simulink model "test_flocking_algorithm"  (R2025b)
settings: Solver=ode4  StartTime=0.0  StopTime=200  FixedStep=0.1  RelTol=1e-3
InitFcn:
  | % initialization_2d
values from neighbouring files (symbols this model uses):
  d2r = 0.0174532925199    [DDPG_HybridFlocking_agents8-4-1.mat]    (also in flocking_learning.m; initialization_2d.m)
  g = spec(2)    [ActualOutput.m]    (also in DDPG_HybridFlocking_agents8-4-1.mat = 9.806; ModelSwarm.m; initialization.m = 9.806; initialization_2d.m = 9.806)
  m = spec(1)    [ActualOutput.m]    (also in DDPG_HybridFlocking_agents8-4-1.mat = 5; ModelSwarm.m; initialization.m = 15; initialization_2d.m = 5)
  state0 = [435.012620465 721.15936685 20 2.59881408791 0 187.945467124 786.05177403 20 2.90689824266 0 842.493878094 376.880931214 ... (25 elements, 5x5)]    [DDPG_HybridFlocking_agents8-4-1.mat]    (also in flocking_learning.m = zeros(5, N); initialization.m = [x0; y0; z0; V0; gam0; psi0]; initialization_2d.m = [x0; y0; V0; psi0; bank0])
undefined symbols (not defined in the file or in its folder): init_state
libraries: simulink_extras x10, rllib x6
(part 1 of 2)
settings Model: Creator=chang  LastModifiedBy=laaa

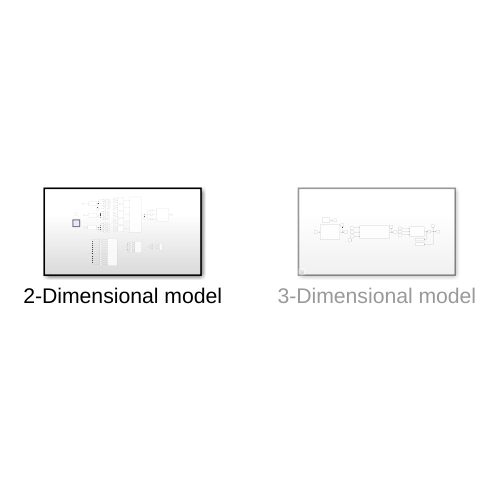
[thumbnail: Simulink's stored preview of the top-level diagram]
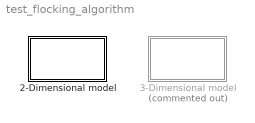
== system test_flocking_algorithm ==
  2-Dimensional model : Subsystem
  3-Dimensional model : Subsystem  Commented=on

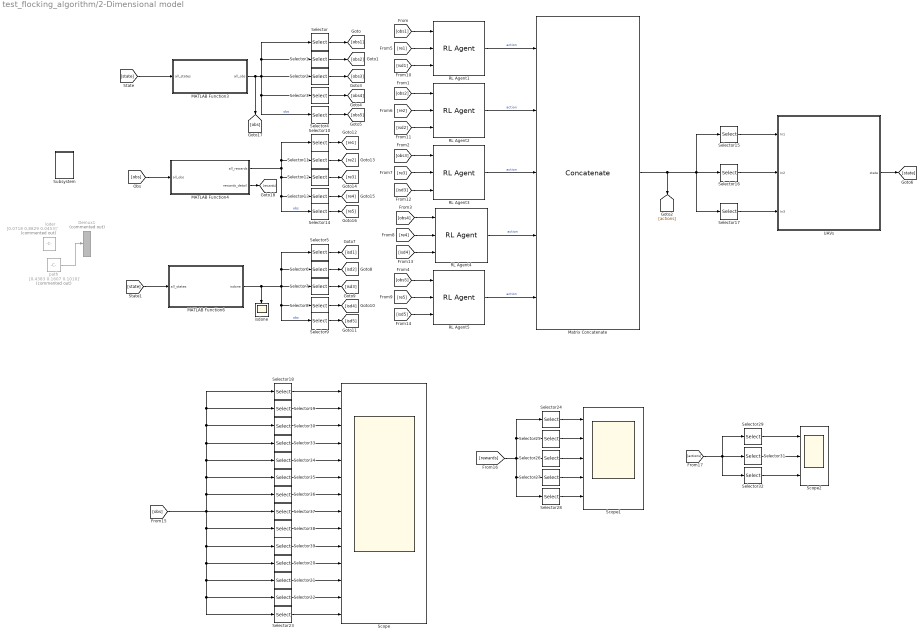
== system test_flocking_algorithm/2-Dimensional model ==
  Demux1 : Demux  Commented=on  Outputs=3
  MATLAB Function3 : MATLAB Function  TreatAsAtomicUnit=on
  MATLAB Function4 : MATLAB Function  TreatAsAtomicUnit=on
  MATLAB Function6 : MATLAB Function  TreatAsAtomicUnit=on
  Matrix Concatenate : Concatenate  NumInputs=5  Mode=Multidimensional array  ConcatenateDimension=2
  RL Agent1 : rllib/RL Agent  Agent=agentObj1  ExternalActionAsInput=off  ProvideLastAction=off  ProvideCumRwd=off  TreatAsDirectFeedthrough=on  UseStrictObservationDataTypes=off
  RL Agent2 : rllib/RL Agent  Agent=agentObj2  ExternalActionAsInput=off  ProvideLastAction=off  ProvideCumRwd=off  TreatAsDirectFeedthrough=on  UseStrictObservationDataTypes=off
  RL Agent3 : rllib/RL Agent  Agent=agentObj3  ExternalActionAsInput=off  ProvideLastAction=off  ProvideCumRwd=off  TreatAsDirectFeedthrough=on  UseStrictObservationDataTypes=off
  RL Agent4 : rllib/RL Agent  Agent=agentObj4  ExternalActionAsInput=off  ProvideLastAction=off  ProvideCumRwd=off  TreatAsDirectFeedthrough=on  UseStrictObservationDataTypes=off
  RL Agent5 : rllib/RL Agent  Agent=agentObj5  ExternalActionAsInput=off  ProvideLastAction=off  ProvideCumRwd=off  TreatAsDirectFeedthrough=on  UseStrictObservationDataTypes=off
  Scope : Scope  NumInputPorts=14
      settings: TimeSpan=200  ActiveDisplayString=12  ShowGrid=off  ActiveDisplayYMinimum=-1.9279504121774151  ActiveDisplayYMaximum=1.9179370597420149  DataLoggingVariableName=ScopeData11
  Scope1 : Scope  NumInputPorts=5
      settings: TimeSpan=200  ActiveDisplayString=5  ShowGrid=off  ActiveDisplayYMinimum=0.0009  ActiveDisplayYMaximum=0.0011  DataLoggingVariableName=ScopeData25
  Scope2 : Scope  NumInputPorts=3
      settings: TimeSpan=200  ActiveDisplayString=3  ShowGrid=off  ActiveDisplayYMinimum=-1  ActiveDisplayYMaximum=1  DataLoggingVariableName=ScopeData26
  Selector : Selector  NumberOfDimensions=2  InputPortWidth=3  IndexOptions=Index vector (dialog),Index vector (dialog)  Indices=1:14,1  OutputSizes=1,1
  Selector1 : Selector  NumberOfDimensions=2  InputPortWidth=3  IndexOptions=Index vector (dialog),Index vector (dialog)  Indices=1:14,2  OutputSizes=1,1
  Selector10 : Selector  NumberOfDimensions=2  InputPortWidth=3  IndexOptions=Index vector (dialog),Index vector (dialog)  Indices=1,1  OutputSizes=1,1
  Selector11 : Selector  NumberOfDimensions=2  InputPortWidth=3  IndexOptions=Index vector (dialog),Index vector (dialog)  Indices=1,2  OutputSizes=1,1
  Selector12 : Selector  NumberOfDimensions=2  InputPortWidth=3  IndexOptions=Index vector (dialog),Index vector (dialog)  Indices=1,3  OutputSizes=1,1
  Selector13 : Selector  NumberOfDimensions=2  InputPortWidth=3  IndexOptions=Index vector (dialog),Index vector (dialog)  Indices=1,4  OutputSizes=1,1
  Selector14 : Selector  NumberOfDimensions=2  InputPortWidth=3  IndexOptions=Index vector (dialog),Index vector (dialog)  Indices=1,5  OutputSizes=1,1
  Selector{15,18,24,29} (4 alike) : Selector  NumberOfDimensions=2  InputPortWidth=3  IndexOptions=Index vector (dialog),Index vector (dialog)  Indices=1,1:5  OutputSizes=1,1
  Selector{16,19,25,31} (4 alike) : Selector  NumberOfDimensions=2  InputPortWidth=3  IndexOptions=Index vector (dialog),Index vector (dialog)  Indices=2,1:5  OutputSizes=1,1
  Selector{17,26,30,32} (4 alike) : Selector  NumberOfDimensions=2  InputPortWidth=3  IndexOptions=Index vector (dialog),Index vector (dialog)  Indices=3,1:5  OutputSizes=1,1
  Selector2 : Selector  NumberOfDimensions=2  InputPortWidth=3  IndexOptions=Index vector (dialog),Index vector (dialog)  Indices=1:14,3  OutputSizes=1,1
  Selector20 : Selector  NumberOfDimensions=2  InputPortWidth=3  IndexOptions=Index vector (dialog),Index vector (dialog)  Indices=11,1:5  OutputSizes=1,1
  Selector21 : Selector  NumberOfDimensions=2  InputPortWidth=3  IndexOptions=Index vector (dialog),Index vector (dialog)  Indices=12,1:5  OutputSizes=1,1
  Selector22 : Selector  NumberOfDimensions=2  InputPortWidth=3  IndexOptions=Index vector (dialog),Index vector (dialog)  Indices=13,1:5  OutputSizes=1,1
  Selector23 : Selector  NumberOfDimensions=2  InputPortWidth=3  IndexOptions=Index vector (dialog),Index vector (dialog)  Indices=14,1:5  OutputSizes=1,1
  Selector27 : Selector  NumberOfDimensions=2  InputPortWidth=3  IndexOptions=Index vector (dialog),Index vector (dialog)  Indices=4,1:5  OutputSizes=1,1
  Selector28 : Selector  NumberOfDimensions=2  InputPortWidth=3  IndexOptions=Index vector (dialog),Index vector (dialog)  Indices=5,1:5  OutputSizes=1,1
  Selector3 : Selector  NumberOfDimensions=2  InputPortWidth=3  IndexOptions=Index vector (dialog),Index vector (dialog)  Indices=1:14,4  OutputSizes=1,1
  Selector33 : Selector  NumberOfDimensions=2  InputPortWidth=3  IndexOptions=Index vector (dialog),Index vector (dialog)  Indices=4,1:5  OutputSizes=1,1
  Selector34 : Selector  NumberOfDimensions=2  InputPortWidth=3  IndexOptions=Index vector (dialog),Index vector (dialog)  Indices=5,1:5  OutputSizes=1,1
  Selector35 : Selector  NumberOfDimensions=2  InputPortWidth=3  IndexOptions=Index vector (dialog),Index vector (dialog)  Indices=6,1:5  OutputSizes=1,1
  Selector36 : Selector  NumberOfDimensions=2  InputPortWidth=3  IndexOptions=Index vector (dialog),Index vector (dialog)  Indices=7,1:5  OutputSizes=1,1
  Selector37 : Selector  NumberOfDimensions=2  InputPortWidth=3  IndexOptions=Index vector (dialog),Index vector (dialog)  Indices=8,1:5  OutputSizes=1,1
  Selector38 : Selector  NumberOfDimensions=2  InputPortWidth=3  IndexOptions=Index vector (dialog),Index vector (dialog)  Indices=9,1:5  OutputSizes=1,1
  Selector39 : Selector  NumberOfDimensions=2  InputPortWidth=3  IndexOptions=Index vector (dialog),Index vector (dialog)  Indices=10,1:5  OutputSizes=1,1
  Selector4 : Selector  NumberOfDimensions=2  InputPortWidth=3  IndexOptions=Index vector (dialog),Index vector (dialog)  Indices=1:14,5  OutputSizes=1,1
  Selector5 : Selector  NumberOfDimensions=2  InputPortWidth=3  IndexOptions=Index vector (dialog),Index vector (dialog)  Indices=1,1  OutputSizes=1,1
  Selector6 : Selector  NumberOfDimensions=2  InputPortWidth=3  IndexOptions=Index vector (dialog),Index vector (dialog)  Indices=1,2  OutputSizes=1,1
  Selector7 : Selector  NumberOfDimensions=2  InputPortWidth=3  IndexOptions=Index vector (dialog),Index vector (dialog)  Indices=1,3  OutputSizes=1,1
  Selector8 : Selector  NumberOfDimensions=2  InputPortWidth=3  IndexOptions=Index vector (dialog),Index vector (dialog)  Indices=1,4  OutputSizes=1,1
  Selector9 : Selector  NumberOfDimensions=2  InputPortWidth=3  IndexOptions=Index vector (dialog),Index vector (dialog)  Indices=1,5  OutputSizes=1,1
  Subsystem : Subsystem
  UAVs : Subsystem
  isdone : Scope
      settings: TimeSpan=300  ActiveDisplayYMinimum=-1  ActiveDisplayYMaximum=1  DataLoggingVariableName=ScopeData23
  loiter : Constant  Commented=on  Value=[0.0718 0.8829 0.0453]'
  path : Constant  Commented=on  Value=[0.4383 0.1607 0.1010]'
  wires:
  Selector4/1 -> [obs5]
  Selector7/1 -> [isd3]
  [re1] -> RL Agent1/2
  [re4] -> RL Agent4/2
  RL Agent1/1 -> Matrix Concatenate/1  "action"
  [isd3] -> RL Agent3/3
  [isd5] -> RL Agent5/3
  RL Agent2/1 -> Matrix Concatenate/2  "action"
  path/1 -> Demux1/1
  [isd2] -> RL Agent2/3
  Selector10/1 -> [re1]
  RL Agent4/1 -> Matrix Concatenate/4  "action"
  Selector17/1 -> UAVs/3(In3)
  Selector8/1 -> [isd4]
  Selector5/1 -> [isd1]
  MATLAB Function6/1(isdone) -> Selector5/1, Selector6/1, Selector7/1, Selector8/1, Selector9/1, isdone/1  "obs"
  [state] -> MATLAB Function6/1(all_states)
  Selector16/1 -> UAVs/2(In2)
  Selector9/1 -> [isd5]
  Selector13/1 -> [re4]
  [obs2] -> RL Agent2/1
  MATLAB Function4/2(rewards_detail) -> [rewards]
  [obs] -> MATLAB Function4/1(all_obs)
  [re3] -> RL Agent3/2
  [obs1] -> RL Agent1/1
  UAVs/1(state) -> [state]
  RL Agent5/1 -> Matrix Concatenate/5  "action"
  Selector3/1 -> [obs4]
  [re2] -> RL Agent2/2
  Selector6/1 -> [isd2]
  [isd1] -> RL Agent1/3
  Selector14/1 -> [re5]
  Selector11/1 -> [re2]
  Selector2/1 -> [obs3]
  MATLAB Function3/1(all_obs) -> Selector2/1, Selector3/1, Selector4/1, Selector/1, Selector1/1, [obs]  "obs"
  Selector1/1 -> [obs2]
  [isd4] -> RL Agent4/3
  Matrix Concatenate/1 -> [actions], Selector16/1, Selector15/1, Selector17/1
  [re5] -> RL Agent5/2
  Selector12/1 -> [re3]
  [obs4] -> RL Agent4/1
  MATLAB Function4/1(all_rewards) -> Selector12/1, Selector13/1, Selector14/1, Selector10/1, Selector11/1  "obs"
  RL Agent3/1 -> Matrix Concatenate/3  "action"
  Selector15/1 -> UAVs/1(In1)
  [obs3] -> RL Agent3/1
  [state] -> MATLAB Function3/1(all_states)
  Selector/1 -> [obs1]
  [obs5] -> RL Agent5/1
  Selector22/1 -> Scope/13
  Selector19/1 -> Scope/2
  Selector36/1 -> Scope/7
  Selector30/1 -> Scope/3
  Selector25/1 -> Scope1/2
  Selector34/1 -> Scope/5
  Selector32/1 -> Scope2/3
  Selector33/1 -> Scope/4
  Selector37/1 -> Scope/8
  Selector26/1 -> Scope1/3
  [actions] -> Selector32/1, Selector29/1, Selector31/1
  Selector38/1 -> Scope/9
  [rewards] -> Selector28/1, Selector27/1, Selector25/1, Selector24/1, Selector26/1
  Selector20/1 -> Scope/11
  Selector24/1 -> Scope1/1
  Selector18/1 -> Scope/1
  [obs] -> Selector39/1, Selector20/1, Selector21/1, Selector23/1, Selector22/1, Selector38/1, Selector33/1, Selector30/1, Selector19/1, Selector18/1, Selector34/1, Selector35/1, Selector36/1, Selector37/1
  Selector23/1 -> Scope/14
  Selector29/1 -> Scope2/1
  Selector27/1 -> Scope1/4
  Selector28/1 -> Scope1/5
  Selector39/1 -> Scope/10
  Selector35/1 -> Scope/6
  Selector31/1 -> Scope2/2
  Selector21/1 -> Scope/12

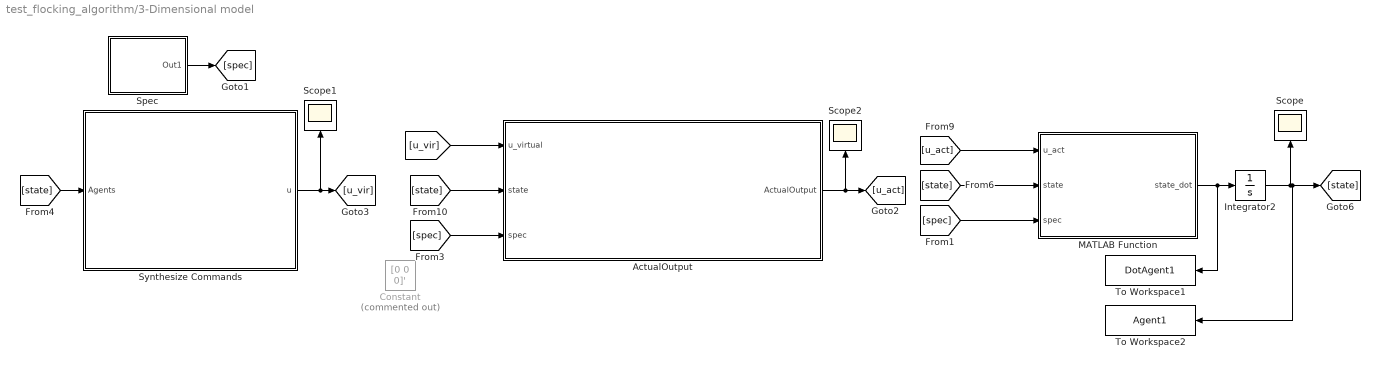
== system test_flocking_algorithm/3-Dimensional model ==
  ActualOutput : Subsystem
  Constant : Constant  Commented=on  Value=[0 0 0]'
  Integrator2 : Integrator  InitialCondition=state0  UpperSaturationLimit=[10^6 ;10^6 ;10^6 ;30 ;15 ;10^6]  LowerSaturationLimit=[-10^6; -10^6 ;-10^6; 0; -15 ;-10^6]'
  MATLAB Function : MATLAB Function  TreatAsAtomicUnit=on
  Scope : Scope
      settings: ActiveDisplayYMinimum=-1796.4442274835574  ActiveDisplayYMaximum=1827.1129411617226
  Scope1 : Scope
      settings: ActiveDisplayYMinimum=-0.625  ActiveDisplayYMaximum=0.625
  Scope2 : Scope
      settings: ActiveDisplayYMinimum=-543.50698903671855  ActiveDisplayYMaximum=2400.6247544411835  DataLoggingVariableName=ScopeData2
  Spec : Subsystem
  Synthesize Commands : Subsystem
  To Workspace1 : ToWorkspace  VariableName=DotAgent1  SaveFormat=Timeseries  SampleTime=-1
  To Workspace2 : ToWorkspace  VariableName=Agent1  SaveFormat=Timeseries  SampleTime=-1
  wires:
  [spec] -> MATLAB Function/3(spec)
  Synthesize Commands/1(u) -> Scope1/1, [u_vir]
  [state] -> ActualOutput/2(state)
  [spec] -> ActualOutput/3(spec)
  [state] -> Synthesize Commands/1(Agents)
  Integrator2/1 -> [state], To Workspace2/1, Scope/1
  [u_vir] -> ActualOutput/1(u_virtual)
  ActualOutput/1(ActualOutput) -> Scope2/1, [u_act]
  MATLAB Function/1(state_dot) -> To Workspace1/1, Integrator2/1
  Spec/1(Out1) -> [spec]
  [state] -> MATLAB Function/2(state)
  [u_act] -> MATLAB Function/1(u_act)

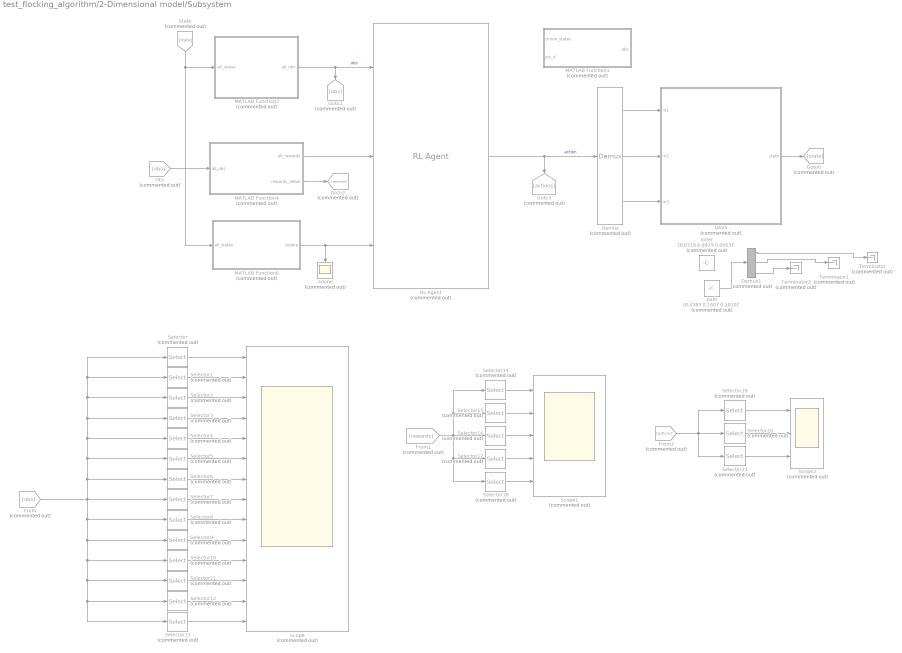
== system test_flocking_algorithm/2-Dimensional model/Subsystem ==
  Demux : Demux  Commented=on  Outputs=3
  Demux1 : Demux  Commented=on  Outputs=3
  From : From  Commented=on  GotoTag=obs
  From1 : From  Commented=on  GotoTag=rewards
  From2 : From  Commented=on  GotoTag=actions
  Goto1 : Goto  Commented=on  GotoTag=obs
  Goto2 : Goto  Commented=on  GotoTag=rewards
  Goto3 : Goto  Commented=on  GotoTag=actions
  Goto6 : Goto  Commented=on  GotoTag=state
  MATLAB Function1 : MATLAB Function  Commented=on  TreatAsAtomicUnit=on
  MATLAB Function3 : MATLAB Function  Commented=on  TreatAsAtomicUnit=on
  MATLAB Function4 : MATLAB Function  Commented=on  TreatAsAtomicUnit=on
  MATLAB Function6 : MATLAB Function  Commented=on  TreatAsAtomicUnit=on
  Obs : From  Commented=on  GotoTag=obs
  RL Agent : rllib/RL Agent  Commented=on  Agent=agent  ExternalActionAsInput=off  ProvideLastAction=off  ProvideCumRwd=off  TreatAsDirectFeedthrough=on  UseStrictObservationDataTypes=off
  Scope : Scope  Commented=on  NumInputPorts=14
      settings: DataLoggingVariableName=ScopeData15
  Scope1 : Scope  Commented=on  NumInputPorts=5
      settings: DataLoggingVariableName=ScopeData17
  Scope2 : Scope  Commented=on  NumInputPorts=3
      settings: DataLoggingVariableName=ScopeData20
  Selector : Selector  Commented=on  NumberOfDimensions=2  InputPortWidth=3  IndexOptions=Index vector (dialog),Index vector (dialog)  Indices=1,1:5  OutputSizes=1,1
  Selector1 : Selector  Commented=on  NumberOfDimensions=2  InputPortWidth=3  IndexOptions=Index vector (dialog),Index vector (dialog)  Indices=2,1:5  OutputSizes=1,1
  Selector10 : Selector  Commented=on  NumberOfDimensions=2  InputPortWidth=3  IndexOptions=Index vector (dialog),Index vector (dialog)  Indices=11,1:5  OutputSizes=1,1
  Selector11 : Selector  Commented=on  NumberOfDimensions=2  InputPortWidth=3  IndexOptions=Index vector (dialog),Index vector (dialog)  Indices=12,1:5  OutputSizes=1,1
  Selector12 : Selector  Commented=on  NumberOfDimensions=2  InputPortWidth=3  IndexOptions=Index vector (dialog),Index vector (dialog)  Indices=13,1:5  OutputSizes=1,1
  Selector13 : Selector  Commented=on  NumberOfDimensions=2  InputPortWidth=3  IndexOptions=Index vector (dialog),Index vector (dialog)  Indices=14,1:5  OutputSizes=1,1
  Selector14 : Selector  Commented=on  NumberOfDimensions=2  InputPortWidth=3  IndexOptions=Index vector (dialog),Index vector (dialog)  Indices=1,1:5  OutputSizes=1,1
  Selector15 : Selector  Commented=on  NumberOfDimensions=2  InputPortWidth=3  IndexOptions=Index vector (dialog),Index vector (dialog)  Indices=2,1:5  OutputSizes=1,1
  Selector16 : Selector  Commented=on  NumberOfDimensions=2  InputPortWidth=3  IndexOptions=Index vector (dialog),Index vector (dialog)  Indices=3,1:5  OutputSizes=1,1
  Selector17 : Selector  Commented=on  NumberOfDimensions=2  InputPortWidth=3  IndexOptions=Index vector (dialog),Index vector (dialog)  Indices=4,1:5  OutputSizes=1,1
  Selector18 : Selector  Commented=on  NumberOfDimensions=2  InputPortWidth=3  IndexOptions=Index vector (dialog),Index vector (dialog)  Indices=5,1:5  OutputSizes=1,1
  Selector19 : Selector  Commented=on  NumberOfDimensions=2  InputPortWidth=3  IndexOptions=Index vector (dialog),Index vector (dialog)  Indices=1,1:5  OutputSizes=1,1
  Selector2 : Selector  Commented=on  NumberOfDimensions=2  InputPortWidth=3  IndexOptions=Index vector (dialog),Index vector (dialog)  Indices=3,1:5  OutputSizes=1,1
  Selector20 : Selector  Commented=on  NumberOfDimensions=2  InputPortWidth=3  IndexOptions=Index vector (dialog),Index vector (dialog)  Indices=2,1:5  OutputSizes=1,1
  Selector21 : Selector  Commented=on  NumberOfDimensions=2  InputPortWidth=3  IndexOptions=Index vector (dialog),Index vector (dialog)  Indices=3,1:5  OutputSizes=1,1
  Selector3 : Selector  Commented=on  NumberOfDimensions=2  InputPortWidth=3  IndexOptions=Index vector (dialog),Index vector (dialog)  Indices=4,1:5  OutputSizes=1,1
  Selector4 : Selector  Commented=on  NumberOfDimensions=2  InputPortWidth=3  IndexOptions=Index vector (dialog),Index vector (dialog)  Indices=5,1:5  OutputSizes=1,1
  Selector5 : Selector  Commented=on  NumberOfDimensions=2  InputPortWidth=3  IndexOptions=Index vector (dialog),Index vector (dialog)  Indices=6,1:5  OutputSizes=1,1
  Selector6 : Selector  Commented=on  NumberOfDimensions=2  InputPortWidth=3  IndexOptions=Index vector (dialog),Index vector (dialog)  Indices=7,1:5  OutputSizes=1,1
  Selector7 : Selector  Commented=on  NumberOfDimensions=2  InputPortWidth=3  IndexOptions=Index vector (dialog),Index vector (dialog)  Indices=8,1:5  OutputSizes=1,1
  Selector8 : Selector  Commented=on  NumberOfDimensions=2  InputPortWidth=3  IndexOptions=Index vector (dialog),Index vector (dialog)  Indices=9,1:5  OutputSizes=1,1
  Selector9 : Selector  Commented=on  NumberOfDimensions=2  InputPortWidth=3  IndexOptions=Index vector (dialog),Index vector (dialog)  Indices=10,1:5  OutputSizes=1,1
  State : From  Commented=on  GotoTag=state
  Terminator : Terminator  Commented=on
  Terminator1 : Terminator  Commented=on
  Terminator2 : Terminator  Commented=on
  UAVs : Subsystem  Commented=on
  isdone : Scope  Commented=on
      settings: TimeSpan=300  ActiveDisplayYMinimum=-1  ActiveDisplayYMaximum=1  DataLoggingVariableName=ScopeData12
  loiter : Constant  Commented=on  Value=[0.0718 0.8829 0.0453]'
  path : Constant  Commented=on  Value=[0.4383 0.1607 0.1010]'
  wires:
  From/1 -> Selector9/1, Selector10/1, Selector11/1, Selector13/1, Selector12/1, Selector8/1, Selector3/1, Selector2/1, Selector1/1, Selector/1, Selector4/1, Selector5/1, Selector6/1, Selector7/1
  Demux/1 -> UAVs/1(In1)
  MATLAB Function3/1(all_obs) -> Goto1/1, RL Agent/1  "obs"
  Selector11/1 -> Scope/12
  Selector10/1 -> Scope/11
  Selector14/1 -> Scope1/1
  Demux/2 -> UAVs/2(In2)
  Obs/1 -> MATLAB Function4/1(all_obs)
  State/1 -> MATLAB Function6/1(all_states), MATLAB Function3/1(all_states)
  From1/1 -> Selector18/1, Selector17/1, Selector15/1, Selector14/1, Selector16/1
  Selector5/1 -> Scope/6
  Selector19/1 -> Scope2/1
  Selector16/1 -> Scope1/3
  Demux1/1 -> Terminator/1
  Selector18/1 -> Scope1/5
  Selector9/1 -> Scope/10
  From2/1 -> Selector21/1, Selector19/1, Selector20/1
  path/1 -> Demux1/1
  RL Agent/1 -> Goto3/1, Demux/1  "action"
  Selector3/1 -> Scope/4
  Selector21/1 -> Scope2/3
  UAVs/1(state) -> Goto6/1
  MATLAB Function6/1(isdone) -> RL Agent/3, isdone/1
  MATLAB Function4/1(all_rewards) -> RL Agent/2
  Selector/1 -> Scope/1
  Demux/3 -> UAVs/3(In3)
  Selector8/1 -> Scope/9
  Selector7/1 -> Scope/8
  Selector6/1 -> Scope/7
  Selector15/1 -> Scope1/2
  Selector2/1 -> Scope/3
  Demux1/3 -> Terminator2/1
  Demux1/2 -> Terminator1/1
  Selector17/1 -> Scope1/4
  Selector20/1 -> Scope2/2
  Selector12/1 -> Scope/13
  Selector13/1 -> Scope/14
  MATLAB Function4/2(rewards_detail) -> Goto2/1
  Selector1/1 -> Scope/2
  Selector4/1 -> Scope/5

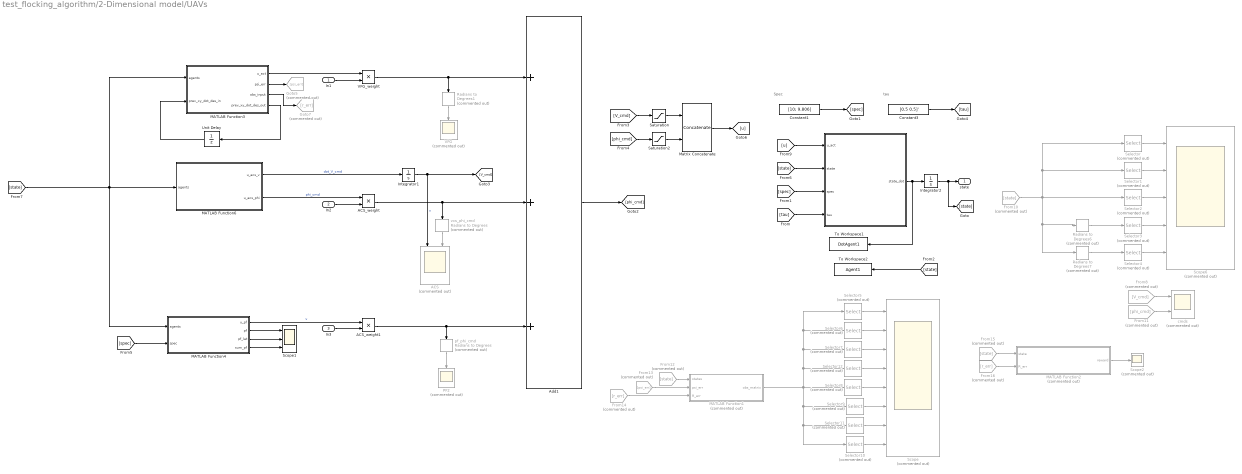
== system test_flocking_algorithm/2-Dimensional model/UAVs ==
  note: Spec
  note: tau
  In1 : Inport
  In2 : Inport  Port=2
  In3 : Inport  Port=3
  " " : MATLAB Function  TreatAsAtomicUnit=on
  ACS : Scope  Commented=on  NumInputPorts=2
      settings: ActiveDisplayYMinimum=-23.869601726691815  ActiveDisplayYMaximum=64.370407175335345  DataLoggingVariableName=ScopeData9
  ACS_weight : Product
  ACS_weight1 : Product
  Add1 : Sum  Inputs=+++
  Constant1 : Constant  Value=[10; 9.806]
  Constant3 : Constant  Value=[0.5 0.5]'
  From10 : From  Commented=on  GotoTag=state
  From11 : From  Commented=on  GotoTag=phi_cmd
  From12 : From  Commented=on  GotoTag=state
  From13 : From  Commented=on  GotoTag=psi_err
  From14 : From  Commented=on  GotoTag=r_err
  From15 : From  Commented=on  GotoTag=state
  From16 : From  Commented=on  GotoTag=r_err
  From8 : From  Commented=on  GotoTag=V_cmd
  Goto5 : Goto  Commented=on  GotoTag=psi_err
  Goto7 : Goto  Commented=on  GotoTag=r_err
  Integrator1 : Integrator  LimitOutput=on  UpperSaturationLimit=35*ones(1,5)  LowerSaturationLimit=15*ones(1,5)
  Integrator2 : Integrator  InitialCondition=init_state  LimitOutput=on  UpperSaturationLimit=[10^6; 10^6; 35; 10^6; 30*d2r ].*ones(1,5)  LowerSaturationLimit=[-10^6; -10^6; 15; -10^6; -30*d2r ].*ones(1,5)
  MATLAB Function1 : MATLAB Function  Commented=on  TreatAsAtomicUnit=on
  MATLAB Function2 : MATLAB Function  Commented=on  TreatAsAtomicUnit=on
  MATLAB Function3 : MATLAB Function  TreatAsAtomicUnit=on
  MATLAB Function4 : MATLAB Function  TreatAsAtomicUnit=on
  MATLAB Function6 : MATLAB Function  TreatAsAtomicUnit=on
  Matrix Concatenate : Concatenate  Mode=Multidimensional array
  PF2 : Scope  Commented=on
      settings: TimeSpan=300  ActiveDisplayYMinimum=-44.741397355611163  ActiveDisplayYMaximum=44.744942341518566  DataLoggingVariableName=ScopeData10
  Radians to Degrees1 : simulink_extras/Transformations/Radians to Degrees  Commented=on
  Radians to Degrees6 : simulink_extras/Transformations/Radians to Degrees  Commented=on
  Radians to Degrees7 : simulink_extras/Transformations/Radians to Degrees  Commented=on
  Saturation : Saturate  UpperLimit=35*ones(1,5)  LowerLimit=15*ones(1,5)
  Saturation2 : Saturate  UpperLimit=30*d2r*ones(1,5)  LowerLimit=-30*d2r*ones(1,5)  LinearizeAsGain=off
  Scope : Scope  Commented=on  NumInputPorts=8
      settings: ActiveDisplayString=4  ActiveDisplayYMinimum=0.29571525373676022  ActiveDisplayYMaximum=1.0782538606959156  DataLoggingVariableName=ScopeData18
  Scope1 : Scope  NumInputPorts=3
      settings: ActiveDisplayYMinimum=-1  ActiveDisplayYMaximum=1  DataLoggingVariableName=ScopeData16
  Scope2 : Scope  Commented=on
      settings: ActiveDisplayYMinimum=-109.38583360755611  ActiveDisplayYMaximum=7.8590338705691378  DataLoggingVariableName=ScopeData19
  Scope6 : Scope  Commented=on  NumInputPorts=5
      settings: TimeSpan=300  ActiveDisplayString=5  ShowGrid=off  ActiveDisplayYMinimum=-37.354494394302066  ActiveDisplayYMaximum=37.435243344907619  YLabel=Bank angle (deg)  DataLoggingVariableName=ScopeData13
  Selector : Selector  Commented=on  NumberOfDimensions=2  InputPortWidth=3  IndexOptions=Index vector (dialog),Index vector (dialog)  Indices=1,1:10  OutputSizes=1,1
  Selector1 : Selector  Commented=on  NumberOfDimensions=2  InputPortWidth=3  IndexOptions=Index vector (dialog),Index vector (dialog)  Indices=2,1:10  OutputSizes=1,1
  Selector10 : Selector  Commented=on  NumberOfDimensions=2  InputPortWidth=3  IndexOptions=Index vector (dialog),Index vector (dialog)  Indices=8,1:5  OutputSizes=1,1
  Selector11 : Selector  Commented=on  NumberOfDimensions=2  InputPortWidth=3  IndexOptions=Index vector (dialog),Index vector (dialog)  Indices=7,1:5  OutputSizes=1,1
  Selector12 : Selector  Commented=on  NumberOfDimensions=2  InputPortWidth=3  IndexOptions=Index vector (dialog),Index vector (dialog)  Indices=4,1:5  OutputSizes=1,1
  Selector2 : Selector  Commented=on  NumberOfDimensions=2  InputPortWidth=3  IndexOptions=Index vector (dialog),Index vector (dialog)  Indices=3,1:10  OutputSizes=1,1
  Selector3 : Selector  Commented=on  NumberOfDimensions=2  InputPortWidth=3  IndexOptions=Index vector (dialog),Index vector (dialog)  Indices=4,1:10  OutputSizes=1,1
  Selector4 : Selector  Commented=on  NumberOfDimensions=2  InputPortWidth=3  IndexOptions=Index vector (dialog),Index vector (dialog)  Indices=5,1:10  OutputSizes=1,1
  Selector5 : Selector  Commented=on  NumberOfDimensions=2  InputPortWidth=3  IndexOptions=Index vector (dialog),Index vector (dialog)  Indices=1,1:5  OutputSizes=1,1
  Selector6 : Selector  Commented=on  NumberOfDimensions=2  InputPortWidth=3  IndexOptions=Index vector (dialog),Index vector (dialog)  Indices=2,1:5  OutputSizes=1,1
  Selector7 : Selector  Commented=on  NumberOfDimensions=2  InputPortWidth=3  IndexOptions=Index vector (dialog),Index vector (dialog)  Indices=3,1:5  OutputSizes=1,1
  Selector8 : Selector  Commented=on  NumberOfDimensions=2  InputPortWidth=3  IndexOptions=Index vector (dialog),Index vector (dialog)  Indices=5,1:5  OutputSizes=1,1
  Selector9 : Selector  Commented=on  NumberOfDimensions=2  InputPortWidth=3  IndexOptions=Index vector (dialog),Index vector (dialog)  Indices=6,1:5  OutputSizes=1,1
  To Workspace1 : ToWorkspace  VariableName=DotAgent1  SaveFormat=Timeseries  SampleTime=-1
  To Workspace2 : ToWorkspace  VariableName=Agent1  SaveFormat=Timeseries  SampleTime=-1
  Unit Delay : UnitDelay  SampleTime=-1  HasFrameUpgradeWarning=on
  VFG : Scope  Commented=on
      settings: ActiveDisplayYMinimum=-2.2311275771009429  ActiveDisplayYMaximum=1.6680942354459041  DataLoggingVariableName=ScopeData8
  VFG_weight : Product
  cmds : Scope  Commented=on  NumInputPorts=2
      settings: ActiveDisplayYMinimum=-0.21104649012249277  ActiveDisplayYMaximum=0.44117626715669322  DataLoggingVariableName=ScopeData14
  pf_phi_cmd : simulink_extras/Transformations/Radians to Degrees  Commented=on
  vcs_phi_cmd : simulink_extras/Transformations/Radians to Degrees  Commented=on
  state : Outport
  wires:
  " "/1(state_dot) -> To Workspace1/1, Integrator2/1
  [state] -> MATLAB Function4/1(agents), MATLAB Function3/1(agents), MATLAB Function6/1(agents)
  [spec] -> MATLAB Function4/2(spec)
  MATLAB Function4/1(u_pf) -> ACS_weight1/1  "v"
  MATLAB Function6/2(u_acs_phi) -> ACS_weight/1  "phi_cmd"
  MATLAB Function3/1(u_act) -> VFG_weight/1
  In1/1 -> VFG_weight/2
  VFG_weight/1 -> Radians to Degrees1/1, Add1/1
  Radians to Degrees1/1 -> VFG/1
  MATLAB Function6/1(u_acs_v) -> Integrator1/1  "dot_V_cmd"
  Integrator1/1 -> ACS/1, [V_cmd]  "v"
  ACS_weight/1 -> Add1/2, vcs_phi_cmd/1
  In2/1 -> ACS_weight/2
  vcs_phi_cmd/1 -> ACS/2
  MATLAB Function4/4(sum_pf) -> Scope1/3
  MATLAB Function4/3(pf_lat) -> Scope1/2
  MATLAB Function4/2(pf) -> Scope1/1
  In3/1 -> ACS_weight1/2
  ACS_weight1/1 -> pf_phi_cmd/1, Add1/3
  pf_phi_cmd/1 -> PF2/1
  Add1/1 -> [phi_cmd]
  [V_cmd] -> Saturation/1
  [phi_cmd] -> Saturation2/1
  Saturation/1 -> Matrix Concatenate/1
  Saturation2/1 -> Matrix Concatenate/2
  Matrix Concatenate/1 -> [u]
  [u] -> " "/1(u_act)
  [state] -> " "/2(state)
  [spec] -> " "/3(spec)
  [tau] -> " "/4(tau)
  Constant1/1 -> [spec]
  Constant3/1 -> [tau]
  Integrator2/1 -> [state], state/1
  [state] -> To Workspace2/1
  Selector/1 -> Scope6/1
  Selector1/1 -> Scope6/2
  Selector2/1 -> Scope6/3
  Selector3/1 -> Scope6/4
  Selector4/1 -> Scope6/5
  From10/1 -> Selector2/1, Selector/1, Selector1/1, Radians to Degrees6/1, Radians to Degrees7/1
  Radians to Degrees6/1 -> Selector3/1
  Radians to Degrees7/1 -> Selector4/1
  From8/1 -> cmds/1
  From11/1 -> cmds/2
  MATLAB Function3/2(psi_err) -> Goto5/1
  MATLAB Function3/3(obs_input) -> Goto7/1
  From12/1 -> MATLAB Function1/1(states)
  From13/1 -> MATLAB Function1/2(psi_err)
  From14/1 -> MATLAB Function1/3(R_err)
  MATLAB Function1/1(obs_matrix) -> Selector6/1, Selector5/1, Selector7/1, Selector12/1, Selector8/1, Selector9/1, Selector10/1, Selector11/1
  Selector9/1 -> Scope/6
  Selector11/1 -> Scope/7
  Selector10/1 -> Scope/8
  Selector5/1 -> Scope/1
  Selector6/1 -> Scope/2
  Selector7/1 -> Scope/3
  Selector12/1 -> Scope/4
  Selector8/1 -> Scope/5
  From15/1 -> MATLAB Function2/1(state)
  From16/1 -> MATLAB Function2/2(R_err)
  MATLAB Function2/1(reward) -> Scope2/1
  MATLAB Function3/4(prev_xy_dot_des_out) -> Unit Delay/1
  Unit Delay/1 -> MATLAB Function3/2(prev_xy_dot_des_in)

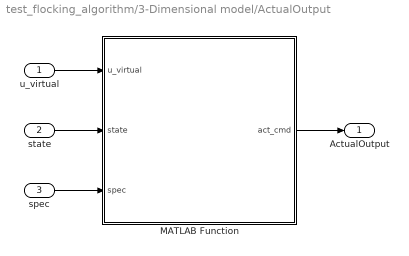
== system test_flocking_algorithm/3-Dimensional model/ActualOutput ==
  u_virtual : Inport
  state : Inport  Port=2
  spec : Inport  Port=3
  MATLAB Function : MATLAB Function  TreatAsAtomicUnit=on
  ActualOutput : Outport
  wires:
  u_virtual/1 -> MATLAB Function/1(u_virtual)
  state/1 -> MATLAB Function/2(state)
  spec/1 -> MATLAB Function/3(spec)
  MATLAB Function/1(act_cmd) -> ActualOutput/1

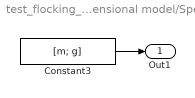
== system test_flocking_algorithm/3-Dimensional model/Spec ==
  Constant3 : Constant  Value=[m; g]
  Out1 : Outport
  wires:
  Constant3/1 -> Out1/1

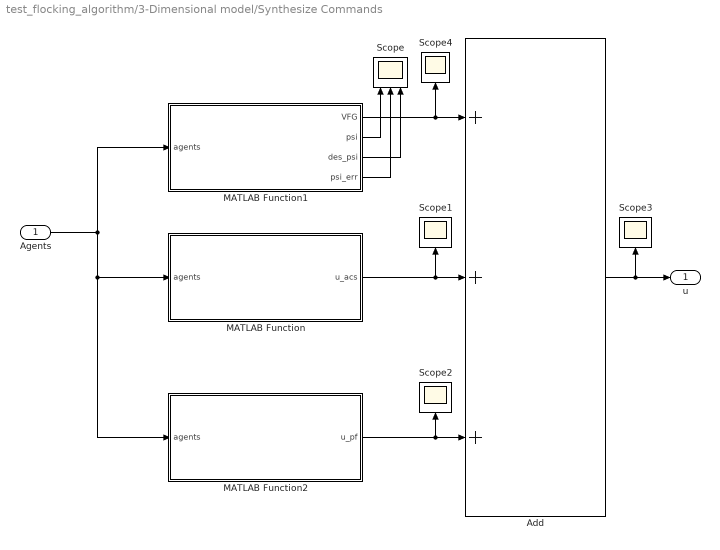
== system test_flocking_algorithm/3-Dimensional model/Synthesize Commands ==
  Agents : Inport
  Add : Sum  Inputs=+++
  MATLAB Function : MATLAB Function  TreatAsAtomicUnit=on
  MATLAB Function1 : MATLAB Function  TreatAsAtomicUnit=on
  MATLAB Function2 : MATLAB Function  TreatAsAtomicUnit=on
  Scope : Scope  NumInputPorts=3
      settings: ActiveDisplayYMinimum=-7.5463075515448264  ActiveDisplayYMaximum=36.500847150660185  DataLoggingVariableName=ScopeData3
  Scope{1..4} (4 alike) : Scope
      Scope1 settings: ActiveDisplayYMinimum=-13.729609129882078  ActiveDisplayYMaximum=15.057455581515576  DataLoggingVariableName=ScopeData4
      Scope2 settings: ActiveDisplayYMinimum=-2.3665763647029392  ActiveDisplayYMaximum=2.4298902475942277  DataLoggingVariableName=ScopeData5
      Scope3 settings: ActiveDisplayYMinimum=-7.2803454393817137  ActiveDisplayYMaximum=5.3802620907689036  DataLoggingVariableName=ScopeData6
      Scope4 settings: ActiveDisplayYMinimum=-15.035450003897875  ActiveDisplayYMaximum=9.9786981173949183  DataLoggingVariableName=ScopeData7
  u : Outport
  wires:
  Agents/1 -> MATLAB Function2/1(agents), MATLAB Function/1(agents), MATLAB Function1/1(agents)
  MATLAB Function1/2(psi) -> Scope/1
  MATLAB Function1/3(des_psi) -> Scope/3
  MATLAB Function1/4(psi_err) -> Scope/2
  MATLAB Function1/1(VFG) -> Add/1, Scope4/1
  MATLAB Function/1(u_acs) -> Scope1/1, Add/2
  MATLAB Function2/1(u_pf) -> Add/3, Scope2/1
  Add/1 -> Scope3/1, u/1

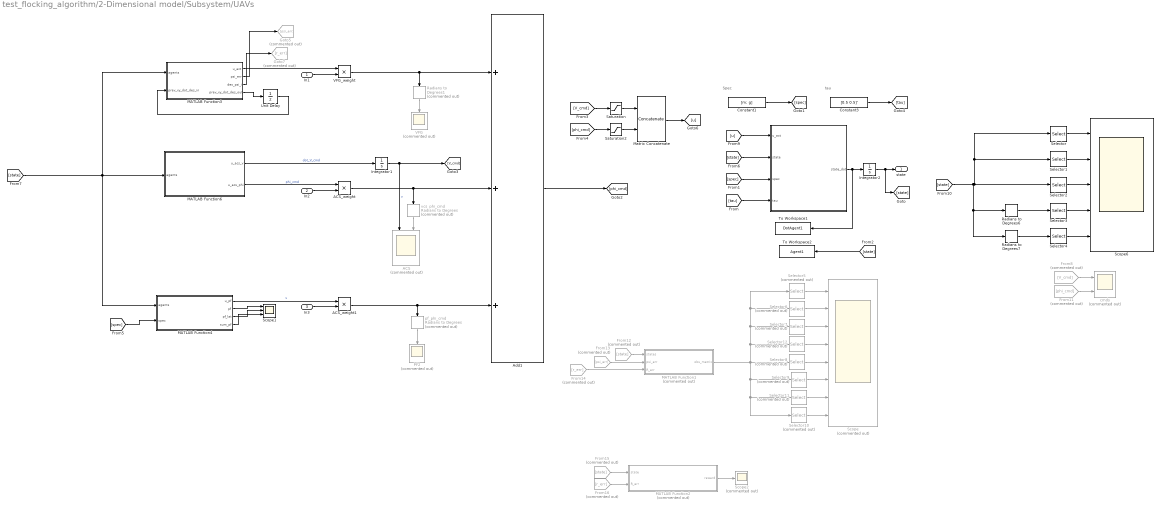
== system test_flocking_algorithm/2-Dimensional model/Subsystem/UAVs ==
  note: Spec
  note: tau
  In1 : Inport
  In2 : Inport  Port=2
  In3 : Inport  Port=3
  " " : MATLAB Function  TreatAsAtomicUnit=on
  ACS : Scope  Commented=on  NumInputPorts=2
      settings: ActiveDisplayYMinimum=-23.869601726691815  ActiveDisplayYMaximum=64.370407175335345  DataLoggingVariableName=ScopeData9
  ACS_weight : Product
  ACS_weight1 : Product
  Add1 : Sum  Inputs=+++
  Constant1 : Constant  Value=[m; g]
  Constant3 : Constant  Value=[0.5 0.5]'
  From11 : From  Commented=on  GotoTag=phi_cmd
  From12 : From  Commented=on  GotoTag=state
  From13 : From  Commented=on  GotoTag=psi_err
  From14 : From  Commented=on  GotoTag=r_err
  From15 : From  Commented=on  GotoTag=state
  From16 : From  Commented=on  GotoTag=r_err
  From8 : From  Commented=on  GotoTag=V_cmd
  Goto5 : Goto  Commented=on  GotoTag=psi_err
  Goto7 : Goto  Commented=on  GotoTag=r_err
  Integrator1 : Integrator  LimitOutput=on  UpperSaturationLimit=35*ones(1,10)  LowerSaturationLimit=15*ones(1,10)
  Integrator2 : Integrator  InitialCondition=state0  LimitOutput=on  UpperSaturationLimit=[10^6; 10^6; 35; 10^6; 30*d2r ]*ones(1,10)  LowerSaturationLimit=[-10^6; -10^6; 15; -10^6; -30*d2r ]*ones(1,10)
  MATLAB Function1 : MATLAB Function  Commented=on  TreatAsAtomicUnit=on
  MATLAB Function2 : MATLAB Function  Commented=on  TreatAsAtomicUnit=on
  MATLAB Function3 : MATLAB Function  TreatAsAtomicUnit=on
  MATLAB Function4 : MATLAB Function  TreatAsAtomicUnit=on
  MATLAB Function6 : MATLAB Function  TreatAsAtomicUnit=on
  Matrix Concatenate : Concatenate  Mode=Multidimensional array
  PF2 : Scope  Commented=on
      settings: TimeSpan=300  ActiveDisplayYMinimum=-44.741397355611163  ActiveDisplayYMaximum=44.744942341518566  DataLoggingVariableName=ScopeData10
  Radians to Degrees1 : simulink_extras/Transformations/Radians to Degrees  Commented=on
  Radians to Degrees6 : simulink_extras/Transformations/Radians to Degrees
  Radians to Degrees7 : simulink_extras/Transformations/Radians to Degrees
  Saturation : Saturate  UpperLimit=35*ones(1,10)  LowerLimit=15*ones(1,10)
  Saturation2 : Saturate  UpperLimit=30*d2r*ones(1,10)  LowerLimit=-30*d2r*ones(1,10)  LinearizeAsGain=off
  Scope : Scope  Commented=on  NumInputPorts=8
      settings: ActiveDisplayString=4  ActiveDisplayYMinimum=0.29571525373676022  ActiveDisplayYMaximum=1.0782538606959156  DataLoggingVariableName=ScopeData18
  Scope1 : Scope  NumInputPorts=3
      settings: ActiveDisplayYMinimum=-1  ActiveDisplayYMaximum=1  DataLoggingVariableName=ScopeData16
  Scope2 : Scope  Commented=on
      settings: ActiveDisplayYMinimum=-109.38583360755611  ActiveDisplayYMaximum=7.8590338705691378  DataLoggingVariableName=ScopeData19
  Scope6 : Scope  NumInputPorts=5
      settings: TimeSpan=300  ActiveDisplayString=5  ShowGrid=off  ActiveDisplayYMinimum=-37.354494394302066  ActiveDisplayYMaximum=37.435243344907619  YLabel=Bank angle (deg)  DataLoggingVariableName=ScopeData13
  Selector : Selector  NumberOfDimensions=2  InputPortWidth=3  IndexOptions=Index vector (dialog),Index vector (dialog)  Indices=1,1:10  OutputSizes=1,1
  Selector1 : Selector  NumberOfDimensions=2  InputPortWidth=3  IndexOptions=Index vector (dialog),Index vector (dialog)  Indices=2,1:10  OutputSizes=1,1
  Selector10 : Selector  Commented=on  NumberOfDimensions=2  InputPortWidth=3  IndexOptions=Index vector (dialog),Index vector (dialog)  Indices=8,1:5  OutputSizes=1,1
  Selector11 : Selector  Commented=on  NumberOfDimensions=2  InputPortWidth=3  IndexOptions=Index vector (dialog),Index vector (dialog)  Indices=7,1:5  OutputSizes=1,1
  Selector12 : Selector  Commented=on  NumberOfDimensions=2  InputPortWidth=3  IndexOptions=Index vector (dialog),Index vector (dialog)  Indices=4,1:5  OutputSizes=1,1
  Selector2 : Selector  NumberOfDimensions=2  InputPortWidth=3  IndexOptions=Index vector (dialog),Index vector (dialog)  Indices=3,1:10  OutputSizes=1,1
  Selector3 : Selector  NumberOfDimensions=2  InputPortWidth=3  IndexOptions=Index vector (dialog),Index vector (dialog)  Indices=4,1:10  OutputSizes=1,1
  Selector4 : Selector  NumberOfDimensions=2  InputPortWidth=3  IndexOptions=Index vector (dialog),Index vector (dialog)  Indices=5,1:10  OutputSizes=1,1
  Selector5 : Selector  Commented=on  NumberOfDimensions=2  InputPortWidth=3  IndexOptions=Index vector (dialog),Index vector (dialog)  Indices=1,1:5  OutputSizes=1,1
  Selector6 : Selector  Commented=on  NumberOfDimensions=2  InputPortWidth=3  IndexOptions=Index vector (dialog),Index vector (dialog)  Indices=2,1:5  OutputSizes=1,1
  Selector7 : Selector  Commented=on  NumberOfDimensions=2  InputPortWidth=3  IndexOptions=Index vector (dialog),Index vector (dialog)  Indices=3,1:5  OutputSizes=1,1
  Selector8 : Selector  Commented=on  NumberOfDimensions=2  InputPortWidth=3  IndexOptions=Index vector (dialog),Index vector (dialog)  Indices=5,1:5  OutputSizes=1,1
  Selector9 : Selector  Commented=on  NumberOfDimensions=2  InputPortWidth=3  IndexOptions=Index vector (dialog),Index vector (dialog)  Indices=6,1:5  OutputSizes=1,1
  To Workspace1 : ToWorkspace  VariableName=DotAgent1  SaveFormat=Timeseries  SampleTime=-1
  To Workspace2 : ToWorkspace  VariableName=Agent1  SaveFormat=Timeseries  SampleTime=-1
  Unit Delay : UnitDelay  SampleTime=-1  HasFrameUpgradeWarning=on
  VFG : Scope  Commented=on
      settings: ActiveDisplayYMinimum=-2.2311275771009429  ActiveDisplayYMaximum=1.6680942354459041  DataLoggingVariableName=ScopeData8
  VFG_weight : Product
  cmds : Scope  Commented=on  NumInputPorts=2
      settings: ActiveDisplayYMinimum=-0.21104649012249277  ActiveDisplayYMaximum=0.44117626715669322  DataLoggingVariableName=ScopeData14
  pf_phi_cmd : simulink_extras/Transformations/Radians to Degrees  Commented=on
  vcs_phi_cmd : simulink_extras/Transformations/Radians to Degrees  Commented=on
  state : Outport
  wires:
  " "/1(state_dot) -> To Workspace1/1, Integrator2/1
  [state] -> MATLAB Function4/1(agents), MATLAB Function3/1(agents), MATLAB Function6/1(agents)
  [spec] -> MATLAB Function4/2(spec)
  MATLAB Function4/1(u_pf) -> ACS_weight1/1  "v"
  MATLAB Function6/2(u_acs_phi) -> ACS_weight/1  "phi_cmd"
  MATLAB Function3/1(u_act) -> VFG_weight/1
  In1/1 -> VFG_weight/2
  VFG_weight/1 -> Add1/1, Radians to Degrees1/1
  Radians to Degrees1/1 -> VFG/1
  MATLAB Function6/1(u_acs_v) -> Integrator1/1  "dot_V_cmd"
  Integrator1/1 -> ACS/1, [V_cmd]  "v"
  ACS_weight/1 -> Add1/2, vcs_phi_cmd/1
  In2/1 -> ACS_weight/2
  vcs_phi_cmd/1 -> ACS/2
  MATLAB Function4/4(sum_pf) -> Scope1/3
  MATLAB Function4/3(pf_lat) -> Scope1/2
  MATLAB Function4/2(pf) -> Scope1/1
  In3/1 -> ACS_weight1/2
  ACS_weight1/1 -> pf_phi_cmd/1, Add1/3
  pf_phi_cmd/1 -> PF2/1
  Add1/1 -> [phi_cmd]
  [V_cmd] -> Saturation/1
  [phi_cmd] -> Saturation2/1
  Saturation/1 -> Matrix Concatenate/1
  Saturation2/1 -> Matrix Concatenate/2
  Matrix Concatenate/1 -> [u]
  [u] -> " "/1(u_act)
  [state] -> " "/2(state)
  [spec] -> " "/3(spec)
  [tau] -> " "/4(tau)
  Constant1/1 -> [spec]
  Constant3/1 -> [tau]
  Integrator2/1 -> [state], state/1
  [state] -> To Workspace2/1
  Selector/1 -> Scope6/1
  Selector1/1 -> Scope6/2
  Selector2/1 -> Scope6/3
  Selector3/1 -> Scope6/4
  Selector4/1 -> Scope6/5
  [state] -> Selector2/1, Selector/1, Selector1/1, Radians to Degrees6/1, Radians to Degrees7/1
  Radians to Degrees6/1 -> Selector3/1
  Radians to Degrees7/1 -> Selector4/1
  From8/1 -> cmds/1
  From11/1 -> cmds/2
  MATLAB Function3/2(psi_err) -> Goto5/1
  MATLAB Function3/3(des_psi_i) -> Goto7/1
  From12/1 -> MATLAB Function1/1(states)
  From13/1 -> MATLAB Function1/2(psi_err)
  From14/1 -> MATLAB Function1/3(R_err)
  MATLAB Function1/1(obs_matrix) -> Selector6/1, Selector5/1, Selector7/1, Selector12/1, Selector8/1, Selector9/1, Selector10/1, Selector11/1
  Selector9/1 -> Scope/6
  Selector11/1 -> Scope/7
  Selector10/1 -> Scope/8
  Selector5/1 -> Scope/1
  Selector6/1 -> Scope/2
  Selector7/1 -> Scope/3
  Selector12/1 -> Scope/4
  Selector8/1 -> Scope/5
  From15/1 -> MATLAB Function2/1(state)
  From16/1 -> MATLAB Function2/2(R_err)
  MATLAB Function2/1(reward) -> Scope2/1
  MATLAB Function3/4(prev_xy_dot_des_out) -> Unit Delay/1
  Unit Delay/1 -> MATLAB Function3/2(prev_xy_dot_des_in)

== matlab function test_flocking_algorithm/2-Dimensional model/Subsystem/MATLAB Function4 ==
  data: all_obs input; all_rewards output; rewards_detail output
function [all_rewards, rewards_detail] = get_reward_normalized(all_obs)
%% get_reward_normalized — 음수 누적형 + Team Reward (협응 학습)
%
%  입력
%   all_obs        : [14 x N]  get_observation_normalized 출력
%
%  출력
%   all_rewards    : [1 x N]   각 에이전트 최종 보상 (개별 + 팀 mix)
%   rewards_detail : [5 x N]   세부 항목 [path; align; flock; col; surv]
%
%  보상 설계
%   r_i_individual = w_p·path_pen + w_a·align_pen + w_f·flock_pen + w_c·col_pen + surv
%   r_i_total      = 0.7 × r_i_individual + 0.3 × mean(r_individual)
%
%  Team mixing 30%의 효과:
%   - 한 명이 다른 명을 R_form 밖으로 밀어내면 자기 보상도 깎임
%   - 자연스러운 협력 압력 → cascade 방지
%   - 30% 비율은 너무 강하지 않게 (개별 학습은 70%로 유지)
%
%  관측 채널 매핑 (14차원에서 추출)
%   obs(1,2) = drel_x, drel_y     (정규화된 R_form 기준)
%   obs(6)   = e_radial           (정규화된 R_orbit 기준)
%   obs(7)   = sin(heading error)
%   obs(11)  = nearest 1 dist / R_safe
%% ------------------------------------------------------------------------

    N              = size(all_obs, 2);
    all_rewards    = zeros(1, N);
    rewards_detail = zeros(5, N);

    %% 채널별 스케일 (gradient 신호 강화)
    s_path  = 0.0125;
    s_align = 0.0075;
    s_flock = 0.0100;
    s_col   = 0.0150;
    surv    = 0.0015;

    %% Team Mixing 비율
    alpha_indiv = 0.7;     % 개별 보상 비중
    alpha_team  = 0.3;     % 팀 평균 보상 비중

    %% 1단계: 각 에이전트의 개별 보상 계산
    individual = zeros(1, N);
    detail     = zeros(5, N);

    for i = 1:N
        obs_i    = all_obs(:, i);
        drel_x   = obs_i(1);
        drel_y   = obs_i(2);
        e_radial = obs_i(6);
        sE       = obs_i(7);
        d_min_n  = obs_i(11);    % nearest 1 distance / R_safe

        % (1) Path error penalty
        path_pen = -s_path * e_radial^2;

        % (2) Align error penalty (heading vs path tangent)
        align_pen = -s_align * sE^2;

        % (3) Flocking penalty (R_form 바깥)
        d_norm    = sqrt(drel_x^2 + drel_y^2);
        excess    = max(0, d_norm - 1);
        flock_pen = -s_flock * excess^2;

        % (4) Collision penalty (R_safe 안)
        danger  = max(0, 1 - d_min_n);
        col_pen = -s_col * danger^2;

        % (5) Survival bonus
        surv_bonus = surv;

        total = path_pen + align_pen + flock_pen + col_pen + surv_bonus;

        % 안전 클램프
        if isnan(total) || isinf(total)
            total = -0.25;
        end
        total = max(min(total, 0.005), -0.5);

        detail(:, i)  = [path_pen; align_pen; flock_pen; col_pen; surv_bonus];
        individual(i) = total;
    end

    %% 2단계: Team Reward Mixing
    team_mean = mean(individual);

    for i = 1:N
        all_rewards(i)       = alpha_indiv * individual(i) + alpha_team * team_mean;
        rewards_detail(:, i) = detail(:, i);    % 디테일은 개별 페널티 그대로 표시
    end
end

== matlab function test_flocking_algorithm/2-Dimensional model/Subsystem/MATLAB Function3 ==
  data: all_obs output size=10; all_states input
function all_obs = get_observation_normalized(all_states)
%% get_observation_normalized — 14차원 벡터화 관측 (k=2 nearest neighbors)
%
%  입력
%   all_states  : [5 x N]  각 열 = (x, y, V, psi, phi)
%  출력
%   all_obs     : [14 x N] 정규화된 관측
%
%  관측 채널 (각 열당 14개)
%   1)  drel_x    = (x_i - x_c)/R_form
%   2)  drel_y    = (y_i - y_c)/R_form
%   3)  dV        = (V_i - V_target)/V_target
%   4)  sin(psi_i)
%   5)  cos(psi_i)
%   6)  e_radial  = (|p_c| - R_orbit)/R_orbit
%   7)  sin(psi_des - psi_i)
%   8)  cos(psi_des - psi_i)
%   9)  Nearest 1: rel_x / R_form
%  10)  Nearest 1: rel_y / R_form
%  11)  Nearest 1: dist  / R_safe
%  12)  Nearest 2: rel_x / R_form
%  13)  Nearest 2: rel_y / R_form
%  14)  Nearest 2: dist  / R_safe
%
%  k=2 이웃 정보를 추가한 이유:
%   - 1개만 보면 "내 옆 친구가 다가오면 멀어짐" → cascade
%   - 2개 보면 "옆 친구가 다가올 때 또 다른 친구가 어디 있는지" 인식
%   - 정책이 "어느 방향으로 비키는 게 안전한지" 학습 가능
%% ------------------------------------------------------------------------

    %% 정규화 상수 (flocking_learning.m 과 동기화)
    R_orbit  = 500;
    V_target = 20;
    R_form   = 75;
    R_safe   = 30;

    N       = size(all_states, 2);
    all_obs = zeros(14, N);

    pos = all_states(1:2, :);
    pc  = mean(pos, 2);

    rc       = norm(pc);
    e_radial = (rc - R_orbit) / R_orbit;
    th_c     = atan2(pc(2), pc(1));
    psi_des  = th_c + pi/2;

    for i = 1:N
        p_i   = pos(:, i);
        V_i   = all_states(3, i);
        psi_i = all_states(4, i);

        % 1,2) 중점 기준 상대 위치
        drel  = (p_i - pc) / R_form;

        % 3) 속도 오차
        dV    = (V_i - V_target) / V_target;

        % 4,5) 헤딩 sin/cos
        sP = sin(psi_i);
        cP = cos(psi_i);

        % 7,8) 접선 방향과 본인 헤딩 차이 (wrap-around 안전)
        dpsi = psi_des - psi_i;
        dpsi = atan2(sin(dpsi), cos(dpsi));
        sE   = sin(dpsi);
        cE   = cos(dpsi);

        % 9-14) 2명의 가장 가까운 이웃
        dists = inf(1, N);
        rels  = zeros(2, N);
        for j = 1:N
            if j == i, continue; end
            rel        = pos(:, j) - p_i;
            dists(j)   = norm(rel);
            rels(:, j) = rel;
        end

        % 거리 오름차순 정렬
        [sorted_d, sorted_idx] = sort(dists);

        % Nearest 1
        if sorted_d(1) < inf
            d1 = sorted_d(1);
            r1 = rels(:, sorted_idx(1));
        else
            d1 = 10 * R_safe;
            r1 = [0; 0];
        end

        % Nearest 2
        if length(sorted_d) >= 2 && sorted_d(2) < inf
            d2 = sorted_d(2);
            r2 = rels(:, sorted_idx(2));
        else
            d2 = 10 * R_safe;
            r2 = [0; 0];
        end

        obs_i = [
            drel(1); drel(2); dV; sP; cP; e_radial; sE; cE;
            r1(1)/R_form; r1(2)/R_form; d1/R_safe;
            r2(1)/R_form; r2(2)/R_form; d2/R_safe
            ];

        % 안전 클램프
        obs_i = max(min(obs_i, 10), -10);
        all_obs(:, i) = obs_i;
    end
end

== matlab function test_flocking_algorithm/2-Dimensional model/Subsystem/MATLAB Function6 ==
  data: all_states input; isdone output
function isdone = check_termination(all_states)
%% check_termination — 벡터화 종료 조건 함수
%  입력
%   all_states : [5 x N]  (x, y, V, psi, phi)
%  출력
%   isdone     : [1 x N]  1 = 해당 에이전트 종료, 0 = 계속
%
%  종료 조건 (어떤 에이전트라도 만족 시 전체 episode 종료)
%   1) 위치가 작업 영역(5km) 밖으로 이탈
%   2) 상태에 NaN/Inf 발생 (수치 폭주)
%   3) 속도가 비정상 범위 (V < 1 m/s 또는 V > 100 m/s)
%
%  Note: 충돌은 종료 조건에 포함하지 않음
%        (보상 함수의 col_pen 으로 연속적으로 학습 신호 부여)
%        → 충돌마다 episode가 끝나면 학습 데이터가 너무 적어짐
%% ------------------------------------------------------------------------

    N      = size(all_states, 2);
    isdone = false(1, N);

    %% 1) 위치 이탈
    pos = all_states(1:2, :);
    out_of_bounds = false;
    for i = 1:N
        if norm(pos(:, i)) > 5000
            out_of_bounds = true;
        end
    end

    %% 2) 수치 폭주
    nan_state = any(any(isnan(all_states))) || any(any(isinf(all_states)));

    %% 3) 비정상 속도
    V    = all_states(3, :);
    bad_V = any(V < 1) || any(V > 100);

    %% 어떤 조건이든 만족 시 모든 에이전트 종료
    if out_of_bounds || nan_state || bad_V
        isdone(:) = true;
    end
end

== matlab function test_flocking_algorithm/2-Dimensional model/Subsystem/UAVs/MATLAB Function3 ==
  data: u_act output; agents input; psi_err output; des_psi_i output; prev_xy_dot_des_in input; prev_xy_dot_des_out output
function [u_act, psi_err, des_psi_i, prev_xy_dot_des_out]  = VFG(agents,prev_xy_dot_des_in)
    % agents: [x; y; V; psi; theta] (5 x N 행렬)
    
    % --- 설정값 ---
    N = size(agents, 2);
    dt = 0.1;
    xt = 0; yt = 0;   
    Vd = 20;          % 드론이 유지해야 할 목표 속도 (m/s)
    rd = 500;         
    g = 9.806;        
    K_vf = 1.5;  
    psi_err = zeros(1,N);
    r_err = zeros(1,N);
    % curr_xy_dot_des_out = zeros(2, N); % 다음 스텝을 위해 밖으로 내보냄
    prev_xy_dot_des_out = zeros(2, N);
    % 출력 변수 초기화 (u_act: 2 x N)
    u_act = zeros(1, N);
    % des_psi = zeros(1, N);
    % psi_err = zeros(1, N);

    for i = 1 : N
        %% 1. 현재 상태 추출
        x = agents(1,i);
        y = agents(2,i);
        V = agents(3,i);      
        psi = agents(4,i);    
        
        %% 2. Vector Field 계산 (Orbit Guidance)
        xr = x - xt;
        yr = y - yt;
        r = sqrt(xr^2 + yr^2);
        r_safe = max(r, 0.1); 
        
        term1 = r_safe^2 - rd^2;
        term2 = 2 * r_safe * rd;
        
        % Vector Field 방향 생성
        xy_dot_dir = [ (term1 * xr + term2 * yr);
                       (term1 * yr - term2 * xr) ];
        
        % 현재 시점의 목표 속도 벡터
        curr_xy_dot_des = -(Vd / (r_safe * (r_safe^2 + rd^2))) * xy_dot_dir;
        % curr_xy_dot_des = xy_dot_dir;
        
        %% 3. 목표 가속도 생성 (수치 미분)
        xy_ddot_des = (curr_xy_dot_des - prev_xy_dot_des_in(:,i)) / dt;
        
        %% 4. 목표 헤딩율(dot_psi_d) 계산
        % N,E_dot
        dot_N = curr_xy_dot_des(1);
        dot_E = curr_xy_dot_des(2);

        % N,E_ddot
        % r_dot = (xr*dot_N + yr*dot_E)/r_safe;
        % ddot_N = dot_N*(r_safe^2-rd^2) - 2*xr*r_safe*r_dot + 2*rd*(dot_E*r_safe + yr*r_dot);
        % ddot_E = dot_E*(r_safe^2-rd^2) - 2*yr*r_safe*r_dot + 2*rd*(dot_N*r_safe + xr*r_dot);
        ddot_N = xy_ddot_des(1);
        ddot_E = xy_ddot_des(2);

        % desired psi
        des_psi_i = atan2(dot_E, dot_N);
        % atan2(sin, cos) 방식이 오차 계산 시 가장 안전합니다.
        % err = atan2(sin(des_psi_i - psi), cos(des_psi_i - psi));
        psi_wrapped = atan2(sin(psi), cos(psi));
        err = des_psi_i - psi_wrapped;
        % [중요] Reddit 로직: 180도(pi)를 넘어가면 반대 방향 최단거리로 보정
        if err > pi
            err = err - 2*pi;
            elseif err < -pi
                err = err + 2*pi;
        end

        psi_err(i) = err;
        r_err(i) = r;


        % desired psi_dot
        vel_sq_safe = max(dot_N^2 + dot_E^2, 0.01); 
        dot_psi_d = (ddot_E * dot_N - dot_E * ddot_N) / vel_sq_safe;
        
        %% 6. 최종 제어 입력 생성 (u_act: 2 x N)
        % 1행: 속도 명령 (멈춰있으면 안 되므로 Vd 또는 현재 V를 넣어줍니다)

        
        % 2행: 뱅크각(Roll) 명령
        u_act(1, i) = atan2(V*(dot_psi_d + K_vf * err), g);
        
        % 결과 저장
        % des_psi(i) = des_psi_i;
        % psi_err(i) = err;
        
        % 상태 업데이트
        prev_xy_dot_des_out(:,i) = curr_xy_dot_des;
    end
end

== matlab function test_flocking_algorithm/2-Dimensional model/Subsystem/UAVs/MATLAB Function4 ==
  data: u_pf output; agents input; spec input; pf output; pf_lat output; sum_pf output
function [u_pf, pf, pf_lat, sum_pf]  = PF(agents, spec)

    %% params
    % idx = 1;
    N = size(agents,2);
    alp = 9; % Potential Strength
    % Bell Function Constant (a, b, c)
    a   = 10; 
    b   = 2;
    c   = 20;
    u_pf = zeros(1,N);
    pf = zeros(1,N);
    denominator = 0;
    sum_pf = zeros(2,N);

    g = spec(2);

    %% Algorithm
    for idx = 1: N
        pos_i = agents(1:2, idx);
        psi = agents(4, idx);
        sum = zeros(2,1);

        for j = 1: N
            if idx==j 
                continue; 
            end
            pos_j = agents(1:2, j);
            pos_ij = pos_i - pos_j;
            pos_ji = pos_j - pos_i;
            norm_ij = norm(pos_ij);
    
            val = (norm_ij - c)/a;
            denominator = 1 + val^(2*b);
            if norm_ij > 0.001
                sum = sum + (alp/denominator)*(pos_ji/norm_ij);
            end
        end
        pf_lat = [-sin(psi) cos(psi)]*[sum(1); sum(2)];
        phi_cmd = atan2(pf_lat, g);
        u_pf(1,idx) = phi_cmd;
        pf(1,idx) = denominator; 
        sum_pf(:,idx) = sum;
    end
end
